simulink library "CAN_lib"  (R2016b)
settings: Solver=VariableStepAuto  StartTime=0.0  StopTime=10.0  RelTol=1e-3
undefined symbols (not defined in the file or in its folder): sim_params
libraries: bus_stubs_fsw x1
settings Model: Creator=taylorreynolds  LastModifiedBy=Taylor

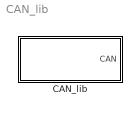
== system CAN_lib ==
  CAN_lib : Subsystem

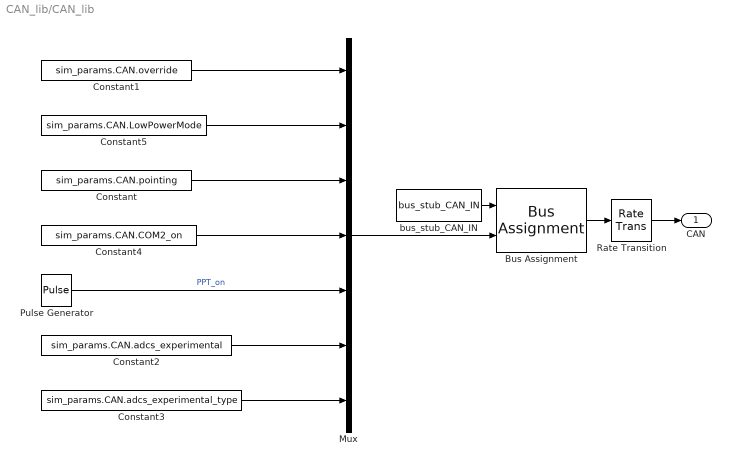
== system CAN_lib/CAN_lib ==
  Bus Assignment : BusAssignment  AssignedSignals=CAN
  Constant : Constant  Value=sim_params.CAN.pointing
  Constant1 : Constant  Value=sim_params.CAN.override
  Constant2 : Constant  Value=sim_params.CAN.adcs_experimental
  Constant3 : Constant  Value=sim_params.CAN.adcs_experimental_type
  Constant4 : Constant  Value=sim_params.CAN.COM2_on
  Constant5 : Constant  Value=sim_params.CAN.LowPowerMode
  Mux : Mux  Inputs=7
  Pulse Generator : DiscretePulseGenerator  PulseType=Time based  Period=sim_params.CAN.sync_pulse_period_s  PulseWidth=sim_params.CAN.PPT_on_sync_pct
  Rate Transition : RateTransition  OutPortSampleTime=sim_params.CAN.sample_time_s
  bus_stub_CAN_IN : bus_stubs_fsw/bus_stub_CAN_IN
  CAN : Outport
  wires:
  Pulse Generator/1 -> Mux/5  "PPT_on"
  Constant/1 -> Mux/3
  Constant1/1 -> Mux/1
  Constant4/1 -> Mux/4
  Constant2/1 -> Mux/6
  Constant3/1 -> Mux/7
  Rate Transition/1 -> CAN/1
  bus_stub_CAN_IN/1 -> Bus Assignment/1
  Bus Assignment/1 -> Rate Transition/1
  Mux/1 -> Bus Assignment/2
  Constant5/1 -> Mux/2
